simulink model "SerialComm"  (R2021a)
settings: Solver=FixedStepAuto  StartTime=0.0  StopTime=10.0  FixedStep=1e-3  RelTol=1e-3  EnableMultiTasking=on
undefined symbols (not defined in the file): A0, A1, D0, D1, D10, D11, D12, D13, D2, D3, D4, D5, D6, D7, D8, D9, magnitude, PTA0, PTA1, PTA2, PTB2, PTB23, PTB3, PTB9, PTC16, PTC17, PTC2, PTC3, PTC4, PTD0, PTD1, PTD2, PTD3
libraries: frdmk64flib x23, etargetslib x6, dspstat3 x1, simulink x1
(part 2 of 3)

== stateflow chart SerialComm/Pacemaker Stateflows ==
  note: Mode selected from DCM changes which State will be run
  state AOO
    entry: Z_VENT_CTRL = false; Z_ATR_CTRL = false; PACING_REF_PWM = AAmplitude;
    VENT_PACE_CTRL = false; VENT_GND_CTRL = false; PACE_GND_CTRL = true;
    note: Charges pacing capacitor and
        | discharges blocking capacitor
    note: Pace Atrium
    note: Duration of Pulse
    state PACE_ATR
      entry:
      PACE_CHARGE_CTRL = false;
      ATR_GND_CTRL = false;
      ATR_PACE_CTRL = true;
      RED_LED = true;
    state C22_CHARGE
      entry:
      PACE_CHARGE_CTRL = true;
      ATR_PACE_CTRL = false;
      ATR_GND_CTRL  = true;
      RED_LED = false;
    note: Wait for LRL before Pulse
    (default) -> AOO.C22_CHARGE
    AOO.PACE_ATR -> AOO.C22_CHARGE : after(APulseW,msec)
    AOO.C22_CHARGE -> AOO.PACE_ATR : after(LRL-uint16(APulseW),msec)
  state MODE_SELECTION
    entry:
    GREEN_LED = false;
    RED_LED = false;
    BLUE_LED = false;
    FRONTEND_CTRL = false;
    PACING_REF_PWM = 0;
    ATR_CMP_REF_PWM = 0;
    VENT_CMP_REF_PWM = 0;
    PACE_CHARGE_CTRL= false;
    PACE_GND_CTRL= false;
    ATR_PACE_CTRL = false;
    ATR_GND_CTRL = false;
    VENT_PACE_CTRL = false;
    VENT_GND_CTRL = false;
    Z_ATR_CTRL = false;
    Z_VENT_CTRL = false;
    note: Reset the values above
        | upon switching modes
  state VOO
    entry: Z_ATR_CTRL = false; Z_VENT_CTRL = false; PACING_REF_PWM = VAmplitude;
    ATR_PACE_CTRL = false; ATR_GND_CTRL = false; PACE_GND_CTRL = true;
    note: Charges pacing capacitor and
        | discharges blocking capacitor
    note: Pace Ventricle
    note: Duration of pulse
    state PACE_VENT
      entry:
      PACE_CHARGE_CTRL = false;
      VENT_GND_CTRL = false;
      VENT_PACE_CTRL = true;
      BLUE_LED = true;
    state C22_CHARGE
      entry:
      VENT_PACE_CTRL = false;
      VENT_GND_CTRL = true;
      PACE_CHARGE_CTRL = true;
      BLUE_LED = false;
    note: Wait for LRL before Pulse
    (default) -> VOO.C22_CHARGE
    VOO.PACE_VENT -> VOO.C22_CHARGE : after(VPulseW,msec)
    VOO.C22_CHARGE -> VOO.PACE_VENT : after(LRL-uint16(VPulseW),msec)
  note: Mode 1
  note: Mode 2
  state AAI
    entry: VENT_PACE_CTRL = false; VENT_GND_CTRL = false; PACE_GND_CTRL = true;
    Z_VENT_CTRL = false; Z_ATR_CTRL = false; FRONTEND_CTRL = true;
    PACING_REF_PWM = AAmplitude; ATR_CMP_REF_PWM=ASensitivity;
    note: Similar to AOO for Pacing
    state PACE_ATR
      entry:
      %discharge C22 capacitor (pacing)
      ATR_PACE_CTRL = true;
      PACE_CHARGE_CTRL = false;
      ATR_GND_CTRL = false;
      RED_LED = true;
    state C22_CHARGE
      entry:
      %discharge C21 capacitor (blocking)
      ATR_PACE_CTRL = false;
      PACE_CHARGE_CTRL = true;
      ATR_GND_CTRL = true;
    state REFRACTORY
      entry: RED_LED = false; PACE_CHARGE_CTRL = true;
      ATR_PACE_CTRL = false;  ATR_GND_CTRL = true;
      exit: GREEN_LED = false;
    note: If a natural pulse is detected, wait ARP period before continuing normal pacing
    (default) -> AAI.C22_CHARGE
    AAI.C22_CHARGE -> AAI.PACE_ATR [order 2] : after(LRL - ARP, msec)
    AAI.C22_CHARGE -> AAI.REFRACTORY [order 1] : [ATR_CMP_DETECT]
        | { GREEN_LED = true; }
    AAI.REFRACTORY -> AAI.C22_CHARGE : after(ARP, msec)
    AAI.PACE_ATR -> AAI.REFRACTORY : after(APulseW, msec)
  state VVI
    entry: ATR_PACE_CTRL = false; ATR_GND_CTRL = false; PACE_GND_CTRL = true;
    Z_VENT_CTRL = false; Z_ATR_CTRL = false; FRONTEND_CTRL = true;
    PACING_REF_PWM = VAmplitude; VENT_CMP_REF_PWM = VSensitivity;
    note: Similar to VOO for Pacing
    state PACE_VENT
      entry:
      %discharge C22 capacitor (pacing)
      PACE_CHARGE_CTRL = false;
      VENT_PACE_CTRL = true;
      VENT_GND_CTRL = false;
      BLUE_LED = true;
    state C22_CHARGE
      entry:
      %discharge C21 capacitor (blocking)
      PACE_CHARGE_CTRL = true;
      VENT_PACE_CTRL = false;
      VENT_GND_CTRL = true;
    state REFRACTORY
      entry: BLUE_LED = false; PACE_CHARGE_CTRL = true;
      VENT_PACE_CTRL = false;  VENT_GND_CTRL = true;
      exit: GREEN_LED = false;
    note: If a natural pulse is detected, wait VRP period before continuing normal pacing
    (default) -> VVI.C22_CHARGE
    VVI.C22_CHARGE -> VVI.PACE_VENT [order 2] : after(LRL - VRP, msec)
    VVI.C22_CHARGE -> VVI.REFRACTORY [order 1] : [VENT_CMP_DETECT]
        | { GREEN_LED = true; }
    VVI.REFRACTORY -> VVI.C22_CHARGE : after(VRP, msec)
    VVI.PACE_VENT -> VVI.REFRACTORY : after(VPulseW, msec)
  note: Mode 3
  note: Mode 4
  state AOOR
    entry:
    Z_VENT_CTRL = false;
    Z_ATR_CTRL = false;
    VENT_PACE_CTRL = false;
    VENT_GND_CTRL = false;
    PACE_GND_CTRL = true;
    PACING_REF_PWM = AAmplitude;
    note: Similar to AOO, but with a dynamic delay for discharging and charging capacitor is provided, calculated in MODULATION
    state PACE [parallel]
      settings: executionOrder=1
      note: Similar to AOO but with rate regulation
      state PACE_ATR
        entry:
        PACE_CHARGE_CTRL = false;
        ATR_GND_CTRL = false;
        ATR_PACE_CTRL = true;
        RED_LED = true;
      state C22_CHARGE
        entry:
        PACE_CHARGE_CTRL = true;
        ATR_PACE_CTRL = false;
        ATR_GND_CTRL = true;
        RED_LED = false;
      (default) -> AOOR.PACE.C22_CHARGE
      AOOR.PACE.PACE_ATR -> AOOR.PACE.C22_CHARGE : after(APulseW,msec)
      AOOR.PACE.C22_CHARGE -> AOOR.PACE.PACE_ATR : after(uint16(ModRate)-uint16(APulseW),msec)
    state MODULATION [parallel]
      entry: increment = double(LRL-MSR)/double(Reaction); decrement = double(LRL - MSR)/double(Recovery);
      during: Target = double(LRL) - (Activity - ActThresh)/double(17 - Response)*2000;
      settings: executionOrder=2
      note: Target dynamically calculates
          | new target throughout the execution
      state STEPUP
        % Decrease delay duration between pulses
        entry: ModRate = ModRate - increment/100;
      note: Clip ModRate
          | to MSR
      note: Clip ModRate
          | to LRL
      state START
        entry:
        ModRate = double(LRL);
      state MAXIMUM
        entry:
        ModRate = double(MSR);
      state STEPDOWN
        % Increase delay duration between pulses
        entry:ModRate = ModRate + decrement/100;
      AOOR.MODULATION.STEPUP -> AOOR.MODULATION.STEPUP [order 2] : after(10,msec)[ModRate > Target]
      AOOR.MODULATION.START -> AOOR.MODULATION.STEPUP : [Target < LRL]
      AOOR.MODULATION.STEPUP -> AOOR.MODULATION.MAXIMUM [order 1] : [ModRate <= MSR]
      AOOR.MODULATION.STEPUP -> AOOR.MODULATION.STEPDOWN [order 3] : after(10,msec)
          | [ModRate <= Target]
      AOOR.MODULATION.STEPDOWN -> AOOR.MODULATION.STEPUP [order 3] : after(10,msec)
          | [ModRate >= Target]
      (default) -> AOOR.MODULATION.START
      AOOR.MODULATION.STEPDOWN -> AOOR.MODULATION.START [order 1] : [ModRate >= LRL]
      AOOR.MODULATION.MAXIMUM -> AOOR.MODULATION.STEPDOWN : [Target > MSR]
      AOOR.MODULATION.STEPDOWN -> AOOR.MODULATION.STEPDOWN [order 2] : after(10, msec)[ModRate < Target]
  state VOOR
    entry:
    ATR_PACE_CTRL = false;
    ATR_GND_CTRL = false;
    PACE_GND_CTRL = true;
    Z_ATR_CTRL = false;
    Z_VENT_CTRL = false;
    PACING_REF_PWM = VAmplitude;
    note: Similar to VOO, but with a dynamic delay for discharging and charging capacitor is provided, calculated in MODULATION
    state PACE [parallel]
      settings: executionOrder=1
      note: Similar to VOO but with rate regulation
      state PACE_VENT
        entry:
        PACE_CHARGE_CTRL = false;
        VENT_GND_CTRL = false;
        VENT_PACE_CTRL = true;
        BLUE_LED = true;
      state C22_CHARGE
        entry:
        VENT_PACE_CTRL = false;
        VENT_GND_CTRL = true;
        PACE_CHARGE_CTRL = true;
        BLUE_LED = false;
      (default) -> VOOR.PACE.C22_CHARGE
      VOOR.PACE.PACE_VENT -> VOOR.PACE.C22_CHARGE : after(VPulseW,msec)
      VOOR.PACE.C22_CHARGE -> VOOR.PACE.PACE_VENT : after(uint16(ModRate)-uint16(VPulseW),msec)
    state MODULATION [parallel]
      entry: increment = double(LRL-MSR)/double(Reaction); decrement = double(LRL - MSR)/double(Recovery);
      during: Target = double(LRL) - (Activity - ActThresh)/double(17 - Response)*2000;
      settings: executionOrder=2
      note: Target dynamically calculates
          | new target throughout the execution
      state STEPUP
        % Decrease delay duration between pulses
        entry: ModRate = ModRate - increment/100;
      note: Clip ModRate
          | to MSR
      note: Clip ModRate
          | to LRL
      state START
        entry:
        ModRate = double(LRL);
      state MAXIMUM
        entry:
        ModRate = double(MSR);
      state STEPDOWN
        % Increase delay duration between pulses
        entry:ModRate = ModRate + decrement/100;
      VOOR.MODULATION.STEPUP -> VOOR.MODULATION.STEPUP [order 2] : after(10,msec)[ModRate > Target]
      VOOR.MODULATION.START -> VOOR.MODULATION.STEPUP : [Target < LRL]
      VOOR.MODULATION.STEPUP -> VOOR.MODULATION.MAXIMUM [order 1] : [ModRate <= MSR]
      VOOR.MODULATION.STEPUP -> VOOR.MODULATION.STEPDOWN [order 3] : after(10,msec)
          | [ModRate <= Target]
      VOOR.MODULATION.STEPDOWN -> VOOR.MODULATION.STEPUP [order 3] : after(10,msec)
          | [ModRate >= Target]
      (default) -> VOOR.MODULATION.START
      VOOR.MODULATION.STEPDOWN -> VOOR.MODULATION.START [order 1] : [ModRate >= LRL]
      VOOR.MODULATION.MAXIMUM -> VOOR.MODULATION.STEPDOWN : [Target > MSR]
      VOOR.MODULATION.STEPDOWN -> VOOR.MODULATION.STEPDOWN [order 2] : after(10, msec)[ModRate < Target]
  note: Mode 5
  note: Mode 6
  state AAIR
    entry: VENT_PACE_CTRL = false; VENT_GND_CTRL = false;  PACE_GND_CTRL = true;
    Z_VENT_CTRL = false; Z_ATR_CTRL = false; FRONTEND_CTRL = true;
    PACING_REF_PWM = AAmplitude; ATR_CMP_REF_PWM=ASensitivity;
    note: Similar to AAI, but with a dynamic delay for discharging and charging capacitor is provided, calculated in MODULATION
    state PACE [parallel]
      settings: executionOrder=1
      state PACE_ATR
        entry:
        ATR_PACE_CTRL = true;
        PACE_CHARGE_CTRL = false;
        ATR_GND_CTRL = false;
        RED_LED = true;
      state C22_CHARGE
        entry:
        ATR_PACE_CTRL = false;
        PACE_CHARGE_CTRL = true;
        ATR_GND_CTRL = true;
      note: Similar to AAI but with Rate Regulation
      state REFRACTORY
        entry: RED_LED = false; PACE_CHARGE_CTRL = true;
        ATR_PACE_CTRL = false;  ATR_GND_CTRL = true;
        exit: GREEN_LED = false;
      (default) -> AAIR.PACE.C22_CHARGE
      AAIR.PACE.C22_CHARGE -> AAIR.PACE.PACE_ATR [order 2] : after(uint16(ModRate) - ARP, msec)
      AAIR.PACE.C22_CHARGE -> AAIR.PACE.REFRACTORY [order 1] : [ATR_CMP_DETECT]
          | { GREEN_LED = true; }
      AAIR.PACE.REFRACTORY -> AAIR.PACE.C22_CHARGE : after(ARP, msec)
      AAIR.PACE.PACE_ATR -> AAIR.PACE.REFRACTORY : after(APulseW, msec)
    state MODULATION [parallel]
      entry: increment = double(LRL-MSR)/double(Reaction); decrement = double(LRL - MSR)/double(Recovery);
      during: Target = double(LRL) - (Activity - ActThresh)/double(17 - Response)*2000;
      settings: executionOrder=2
      note: Target dynamically calculates
          | new target throughout the execution
      state STEPUP
        % Decrease delay duration between pulses
        entry: ModRate = ModRate - increment/100;
      note: Clip ModRate
          | to MSR
      note: Clip ModRate
          | to LRL
      state START
        entry:
        ModRate = double(LRL);
      state MAXIMUM
        entry:
        ModRate = double(MSR);
      state STEPDOWN
        % Increase delay duration between pulses
        entry:ModRate = ModRate + decrement/100;
      AAIR.MODULATION.STEPUP -> AAIR.MODULATION.STEPUP [order 2] : after(10,msec)[ModRate > Target]
      AAIR.MODULATION.START -> AAIR.MODULATION.STEPUP : [Target < LRL]
      AAIR.MODULATION.STEPUP -> AAIR.MODULATION.MAXIMUM [order 1] : [ModRate <= MSR]
      AAIR.MODULATION.STEPUP -> AAIR.MODULATION.STEPDOWN [order 3] : after(10,msec)
          | [ModRate <= Target]
      AAIR.MODULATION.STEPDOWN -> AAIR.MODULATION.STEPUP [order 3] : after(10,msec)
          | [ModRate >= Target]
      (default) -> AAIR.MODULATION.START
      AAIR.MODULATION.STEPDOWN -> AAIR.MODULATION.START [order 1] : [ModRate >= LRL]
      AAIR.MODULATION.MAXIMUM -> AAIR.MODULATION.STEPDOWN : [Target > MSR]
      AAIR.MODULATION.STEPDOWN -> AAIR.MODULATION.STEPDOWN [order 2] : after(10, msec)[ModRate < Target]
  state VVIR
    entry: ATR_PACE_CTRL = false; ATR_GND_CTRL = false; PACE_GND_CTRL = true;
    Z_VENT_CTRL = false; Z_ATR_CTRL = false; FRONTEND_CTRL = true;
    PACING_REF_PWM = VAmplitude; VENT_CMP_REF_PWM = VSensitivity;
    note: Similar to VVI, but with a dynamic delay for discharging and charging capacitor is provided, calculated in MODULATION
    state PACE [parallel]
      settings: executionOrder=1
      state PACE_VENT
        entry:
        PACE_CHARGE_CTRL = false;
        VENT_PACE_CTRL = true;
        VENT_GND_CTRL = false;
        BLUE_LED = true;
      state C22_CHARGE
        entry:
        PACE_CHARGE_CTRL = true;
        VENT_PACE_CTRL = false;
        VENT_GND_CTRL = true;
      state REFRACTORY
        entry: BLUE_LED = false; PACE_CHARGE_CTRL = true;
        VENT_PACE_CTRL = false;  VENT_GND_CTRL = true;
        exit: GREEN_LED = false;
      note: Similar to VVI but with rate regulation
      (default) -> VVIR.PACE.C22_CHARGE
      VVIR.PACE.C22_CHARGE -> VVIR.PACE.PACE_VENT [order 2] : after(uint16(ModRate)-VRP,msec)
      VVIR.PACE.C22_CHARGE -> VVIR.PACE.REFRACTORY [order 1] : [VENT_CMP_DETECT]
          | { GREEN_LED = true; }
      VVIR.PACE.REFRACTORY -> VVIR.PACE.C22_CHARGE : after(VRP, msec)
      VVIR.PACE.PACE_VENT -> VVIR.PACE.REFRACTORY : after(VPulseW, msec)
    state MODULATION [parallel]
      entry: increment = double(LRL-MSR)/double(Reaction); decrement = double(LRL - MSR)/double(Recovery);
      during: Target = double(LRL) - (Activity - ActThresh)/double(17 - Response)*2000;
      settings: executionOrder=2
      note: Target dynamically calculates
          | new target throughout the execution
      state STEPUP
        % Decrease delay duration between pulses
        entry: ModRate = ModRate - increment/100;
      note: Clip ModRate
          | to MSR
      note: Clip ModRate
          | to LRL
      state START
        entry:
        ModRate = double(LRL);
      state MAXIMUM
        entry:
        ModRate = double(MSR);
      state STEPDOWN
        % Increase delay duration between pulses
        entry:ModRate = ModRate + decrement/100;
      VVIR.MODULATION.STEPUP -> VVIR.MODULATION.STEPUP [order 2] : after(10,msec)[ModRate > Target]
      VVIR.MODULATION.START -> VVIR.MODULATION.STEPUP : [Target < LRL]
      VVIR.MODULATION.STEPUP -> VVIR.MODULATION.MAXIMUM [order 1] : [ModRate <= MSR]
      VVIR.MODULATION.STEPUP -> VVIR.MODULATION.STEPDOWN [order 3] : after(10,msec)
          | [ModRate <= Target]
      VVIR.MODULATION.STEPDOWN -> VVIR.MODULATION.STEPUP [order 3] : after(10,msec)
          | [ModRate >= Target]
      (default) -> VVIR.MODULATION.START
      VVIR.MODULATION.STEPDOWN -> VVIR.MODULATION.START [order 1] : [ModRate >= LRL]
      VVIR.MODULATION.MAXIMUM -> VVIR.MODULATION.STEPDOWN : [Target > MSR]
      VVIR.MODULATION.STEPDOWN -> VVIR.MODULATION.STEPDOWN [order 2] : after(10, msec)[ModRate < Target]
  note: Mode 7
  note: Mode 8
  state DOO
    entry: Z_VENT_CTRL = false; Z_ATR_CTRL = false; PACE_GND_CTRL = true;
    note: Charge Pacing Capacitor,
        | discharge Blocking Capacitor,
        | for Atrium
    note: Pace Atrium
    state C22_CHARGE
      entry:
      ATR_PACE_CTRL = false;
      VENT_PACE_CTRL = false;
      PACING_REF_PWM = AAmplitude;
      PACE_CHARGE_CTRL = true;
      ATR_GND_CTRL = false;
      VENT_GND_CTRL = true;
      BLUE_LED = false;
    state PACE_ATR
      entry:
      PACE_CHARGE_CTRL = false;
      ATR_GND_CTRL = false;
      VENT_GND_CTRL = false;
      ATR_PACE_CTRL = true;
      RED_LED = true;
    note: Duration of Atrium pulse
    state AVDelay_PERIOD
      entry:
      ATR_PACE_CTRL = false;
      VENT_PACE_CTRL = false;
      PACING_REF_PWM = VAmplitude;
      PACE_CHARGE_CTRL = true;
      ATR_GND_CTRL = true;
      VENT_GND_CTRL = false;
      RED_LED = false;
    note: Duration of Ventricle Pulse
    state PACE_VENT
      entry:
      PACE_CHARGE_CTRL = false;
      ATR_GND_CTRL = false;
      VENT_GND_CTRL = false;
      VENT_PACE_CTRL = true;
      BLUE_LED = true;
    note: Pace Ventricle
    note: Charge Pacing Capacitor, discharge
        | Blocking Capacitor, for Atrium
    (default) -> DOO.C22_CHARGE
    DOO.C22_CHARGE -> DOO.PACE_ATR : after(LRL-AVDelay-uint16(VPulseW),msec)
    DOO.PACE_ATR -> DOO.AVDelay_PERIOD : after(APulseW,msec)
    DOO.PACE_VENT -> DOO.C22_CHARGE : after(VPulseW, msec)
    DOO.AVDelay_PERIOD -> DOO.PACE_VENT : after(AVDelay-uint16(APulseW),msec)
  state DOOR
    entry: Z_VENT_CTRL = false; Z_ATR_CTRL = false; PACE_GND_CTRL = true;
    note: Similar to DOO, but with Rate Regulation
    state Pace [parallel]
      settings: executionOrder=1
      note: Charge Pacing Capacitor,
          | discharge Blocking Capacitor,
          | for Atrium
      note: Pace Atrium
      state PACE_ATR
        entry:
        PACE_CHARGE_CTRL = false;
        ATR_GND_CTRL = false;
        VENT_GND_CTRL = false;
        ATR_PACE_CTRL = true;
        RED_LED = true;
      state C22_CHARGE
        entry:
        ATR_PACE_CTRL = false;
        VENT_PACE_CTRL = false;
        PACING_REF_PWM = AAmplitude;
        PACE_CHARGE_CTRL = true;
        ATR_GND_CTRL = false;
        VENT_GND_CTRL = true;
        BLUE_LED = false;
      note: Duration of Atrium pulse
      state AVDelay_PERIOD
        entry:
        ATR_PACE_CTRL = false;
        VENT_PACE_CTRL = false;
        PACING_REF_PWM = VAmplitude;
        PACE_CHARGE_CTRL = true;
        ATR_GND_CTRL = true;
        VENT_GND_CTRL = false;
        RED_LED = false;
      note: Duration of Ventricle Pulse
      state PACE_VENT
        entry:
        PACE_CHARGE_CTRL = false;
        ATR_GND_CTRL = false;
        VENT_GND_CTRL = false;
        VENT_PACE_CTRL = true;
        BLUE_LED = true;
      note: Pace Ventricle
      note: Charge Pacing Capacitor, discharge
          | Blocking Capacitor, for Atrium
      (default) -> DOOR.Pace.C22_CHARGE
      DOOR.Pace.C22_CHARGE -> DOOR.Pace.PACE_ATR : after(uint16(ModRate)-AVDelay-uint16(VPulseW),msec)
      DOOR.Pace.PACE_ATR -> DOOR.Pace.AVDelay_PERIOD : after(APulseW,msec)
      DOOR.Pace.PACE_VENT -> DOOR.Pace.C22_CHARGE : after(VPulseW, msec)
      DOOR.Pace.AVDelay_PERIOD -> DOOR.Pace.PACE_VENT : after(AVDelay-uint16(APulseW),msec)
    state MODULATION [parallel]
      entry: increment = double(LRL-MSR)/double(Reaction); decrement = double(LRL - MSR)/double(Recovery);
      during: Target = double(LRL) - (Activity - ActThresh)/double(17 - Response)*2000;
      settings: executionOrder=2
      note: Target dynamically calculates
          | new target throughout the execution
      state STEPUP
        % Decrease delay duration between pulses
        entry: ModRate = ModRate - increment/100;
      note: Clip ModRate
          | to MSR
      note: Clip ModRate
          | to LRL
      state START
        entry:
        ModRate = double(LRL);
      state MAXIMUM
        entry:
        ModRate = double(MSR);
      state STEPDOWN
        % Increase delay duration between pulses
        entry:ModRate = ModRate + decrement/100;
      DOOR.MODULATION.STEPUP -> DOOR.MODULATION.STEPUP [order 2] : after(10,msec)[ModRate > Target]
      DOOR.MODULATION.START -> DOOR.MODULATION.STEPUP : [Target < LRL]
      DOOR.MODULATION.STEPUP -> DOOR.MODULATION.MAXIMUM [order 1] : [ModRate <= MSR]
      DOOR.MODULATION.STEPUP -> DOOR.MODULATION.STEPDOWN [order 3] : after(10,msec)
          | [ModRate <= Target]
      DOOR.MODULATION.STEPDOWN -> DOOR.MODULATION.STEPUP [order 3] : after(10,msec)
          | [ModRate >= Target]
      (default) -> DOOR.MODULATION.START
      DOOR.MODULATION.STEPDOWN -> DOOR.MODULATION.START [order 1] : [ModRate >= LRL]
      DOOR.MODULATION.MAXIMUM -> DOOR.MODULATION.STEPDOWN : [Target > MSR]
      DOOR.MODULATION.STEPDOWN -> DOOR.MODULATION.STEPDOWN [order 2] : after(10, msec)[ModRate < Target]
  state DDD
    entry: Z_VENT_CTRL = false; Z_ATR_CTRL = false; PACE_GND_CTRL = true;
    during: ATR_CMP_REF_PWM = ASensitivity; VENT_CMP_REF_PWM = VSensitivity;
    state PACE_ATR
      entry:
      PACE_CHARGE_CTRL = false;
      ATR_GND_CTRL = false;
      VENT_GND_CTRL = false;
      ATR_PACE_CTRL = true;
      RED_LED = true;
    state C22_CHARGE
      entry:
      ATR_PACE_CTRL = false;
      VENT_PACE_CTRL = false;
      PACING_REF_PWM = AAmplitude;
      PACE_CHARGE_CTRL = true;
      ATR_GND_CTRL = false;
      VENT_GND_CTRL = true;
      BLUE_LED = false;
      GREEN_LED = false;
    state AVDelay_PERIOD
      entry:
      ATR_PACE_CTRL = false;
      VENT_PACE_CTRL = false;
      PACING_REF_PWM = VAmplitude;
      PACE_CHARGE_CTRL = true;
      ATR_GND_CTRL = true;
      VENT_GND_CTRL = false;
      RED_LED = false;
    state PACE_VENT
      entry:
      PACE_CHARGE_CTRL = false;
      ATR_GND_CTRL = false;
      VENT_GND_CTRL = false;
      VENT_PACE_CTRL = true;
      BLUE_LED = true;
    (default) -> DDD.C22_CHARGE
    DDD.C22_CHARGE -> DDD.PACE_ATR [order 2] : after(LRL-AVDelay-uint16(VPulseW),msec)
    DDD.PACE_ATR -> DDD.AVDelay_PERIOD : after(APulseW,msec)
    DDD.C22_CHARGE -> DDD.AVDelay_PERIOD [order 1] : after(APulseW,msec)
        | [ATR_CMP_DETECT]
    DDD.AVDelay_PERIOD -> DDD.C22_CHARGE [order 1] : after(APulseW,msec)
        | [VENT_CMP_DETECT]
    DDD.PACE_VENT -> DDD.C22_CHARGE : after(VPulseW,msec)
    DDD.AVDelay_PERIOD -> DDD.PACE_VENT [order 2] : after(AVDelay-uint16(APulseW),msec)
  state DDDR
    entry: Z_VENT_CTRL = false; Z_ATR_CTRL = false; PACE_GND_CTRL = true;
    during: ATR_CMP_REF_PWM=ASensitivity; VENT_CMP_REF_PWM = VSensitivity;
    state Pace [parallel]
      settings: executionOrder=1
      note: This is "DDD"
      state PACE_ATR
        entry:
        PACE_CHARGE_CTRL = false;
        ATR_GND_CTRL = false;
        VENT_GND_CTRL = false;
        ATR_PACE_CTRL = true;
        RED_LED = true;
      state C22_CHARGE
        entry:
        ATR_PACE_CTRL = false;
        VENT_PACE_CTRL = false;
        PACING_REF_PWM = AAmplitude;
        PACE_CHARGE_CTRL = true;
        ATR_GND_CTRL = false;
        VENT_GND_CTRL = true;
        BLUE_LED = false;
      state AVDelay_PERIOD
        entry:
        ATR_PACE_CTRL = false;
        VENT_PACE_CTRL = false;
        PACING_REF_PWM = VAmplitude;
        PACE_CHARGE_CTRL = true;
        ATR_GND_CTRL = true;
        VENT_GND_CTRL = false;
        RED_LED = false;
      state PACE_VENT
        entry:
        PACE_CHARGE_CTRL = false;
        ATR_GND_CTRL = false;
        VENT_GND_CTRL = false;
        VENT_PACE_CTRL = true;
        BLUE_LED = true;
      (default) -> DDDR.Pace.C22_CHARGE
      DDDR.Pace.C22_CHARGE -> DDDR.Pace.PACE_ATR [order 2] : after(uint16(ModRate)-AVDelay-uint16(VPulseW),msec)
      DDDR.Pace.C22_CHARGE -> DDDR.Pace.AVDelay_PERIOD [order 1] : after(APulseW,msec)
          | [ATR_CMP_DETECT]
      DDDR.Pace.PACE_ATR -> DDDR.Pace.AVDelay_PERIOD : after(APulseW,msec)
      DDDR.Pace.AVDelay_PERIOD -> DDDR.Pace.C22_CHARGE [order 1] : after(VPulseW,msec)
          | [VENT_CMP_DETECT]
      DDDR.Pace.PACE_VENT -> DDDR.Pace.C22_CHARGE : after(VPulseW, msec)
      DDDR.Pace.AVDelay_PERIOD -> DDDR.Pace.PACE_VENT [order 2] : after(AVDelay-uint16(APulseW),msec)
    state MODULATION [parallel]
      during: increment = double(LRL-MSR)/double(Reaction); decrement = double(LRL - MSR)/double(Recovery);
      Target = double(LRL) - (Activity - ActThresh)/double(17 - Response)*2000;
      settings: executionOrder=2
      note: Target dynamically calculates
          | new target throughout the execution
      state STEPUP
        % Decrease delay duration between pulses
        entry: ModRate = ModRate - increment/100;
      note: Clip ModRate
          | to MSR
      note: Clip ModRate
          | to LRL
      state START
        entry:
        ModRate = double(LRL);
      state MAXIMUM
        entry:
        ModRate = double(MSR);
      state STEPDOWN
        % Increase delay duration between pulses
        entry:ModRate = ModRate + decrement/100;
      DDDR.MODULATION.STEPUP -> DDDR.MODULATION.STEPUP [order 2] : after(10,msec)[ModRate > Target]
      DDDR.MODULATION.START -> DDDR.MODULATION.STEPUP : [Target < LRL]
      DDDR.MODULATION.STEPUP -> DDDR.MODULATION.MAXIMUM [order 1] : [ModRate <= MSR]
      DDDR.MODULATION.STEPUP -> DDDR.MODULATION.STEPDOWN [order 3] : after(10,msec)
          | [ModRate <= Target]
      DDDR.MODULATION.STEPDOWN -> DDDR.MODULATION.STEPUP [order 3] : after(10,msec)
          | [ModRate >= Target]
      (default) -> DDDR.MODULATION.START
      DDDR.MODULATION.STEPDOWN -> DDDR.MODULATION.START [order 1] : [ModRate >= LRL]
      DDDR.MODULATION.MAXIMUM -> DDDR.MODULATION.STEPDOWN : [Target > MSR]
      DDDR.MODULATION.STEPDOWN -> DDDR.MODULATION.STEPDOWN [order 2] : after(10, msec)[ModRate < Target]
  note: Mode 9
  note: Mode 10
  note: Mode 11
  note: Mode 12
  (default) -> MODE_SELECTION
  MODE_SELECTION -> VOO [order 2] : [Mode==2]
  MODE_SELECTION -> AOO [order 1] : [Mode==1]
  VOO -> MODE_SELECTION : [Mode~=2]
  AOO -> MODE_SELECTION : [Mode~=1]
  MODE_SELECTION -> AAI [order 3] : [Mode==3]
  MODE_SELECTION -> VVI [order 4] : [Mode==4]
  AAI -> MODE_SELECTION : [Mode~=3]
  VVI -> MODE_SELECTION : [Mode~=4]
  MODE_SELECTION -> AOOR [order 5] : [Mode==5]
  MODE_SELECTION -> VOOR [order 6] : [Mode==6]
  AOOR -> MODE_SELECTION : [Mode~=5]
  VOOR -> MODE_SELECTION : [Mode~=6]
  MODE_SELECTION -> VVIR [order 8] : [Mode==8]
  MODE_SELECTION -> AAIR [order 7] : [Mode==7]
  AAIR -> MODE_SELECTION : [Mode~=7]
  VVIR -> MODE_SELECTION : [Mode~=8]
  MODE_SELECTION -> DOO [order 9] : [Mode==9]
  DOO -> MODE_SELECTION : [Mode~=9]
  MODE_SELECTION -> DOOR [order 10] : [Mode==10]
  DOOR -> MODE_SELECTION : [Mode~=10]
  DDD -> MODE_SELECTION : [Mode~=11]
  MODE_SELECTION -> DDD [order 11] : [Mode==11]
  DDDR -> MODE_SELECTION : [Mode~=12]
  MODE_SELECTION -> DDDR [order 12] : [Mode==12]
  data: LRL input uint16; AAmplitude input uint8; APulseW input uint8; ASensitivity input uint8; ARP input uint16; VAmplitude input uint8; VPulseW input uint8; VSensitivity input uint8; VRP input uint16; Reaction input uint8; ActThresh input double; Response input uint8; PACE_CHARGE_CTRL output boolean; VENT_CMP_REF_PWM output uint8; Z_ATR_CTRL output boolean; PACING_REF_PWM output uint8; ATR_CMP_REF_PWM output uint8; Z_VENT_CTRL output boolean; ATR_PACE_CTRL output boolean; VENT_PACE_CTRL output boolean; PACE_GND_CTRL output boolean; ATR_GND_CTRL output boolean; VENT_GND_CTRL output boolean; Mode input uint8; Recovery input uint16; FRONTEND_CTRL output boolean; RED_LED output boolean; GREEN_LED output boolean; BLUE_LED output boolean; ATR_CMP_DETECT input boolean; VENT_CMP_DETECT input boolean; AVDelay input uint16; Activity input double; ModRate local double; MSR input uint16; Target local double; decrement local double; increment local double
